simulink model "sfcndemo_port_triggered"  (Simulink 6.0)
settings: Solver=FixedStepDiscrete  SolverMode=SingleTasking  StartTime=0.0  StopTime=10.0  RelTol=1e-3
settings Model: Creator=The MathWorks Inc.  LastModifiedBy=batserve  ExtModeAutoUpdateStatusClock=off
settings OptimizationCC: BooleanDataType=off  InlineInvariantSignals=off
settings DebuggingCC: CheckExecutionContextPreStartOutputMsg=on  CheckExecutionContextRuntimeOutputMsg=on  SolverPrmCheckMsg=none
settings HardwareCC: TargetUnknown=on

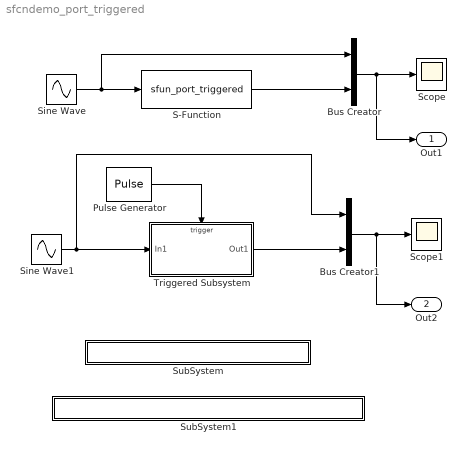
== system sfcndemo_port_triggered ==
  Bus Creator : BusCreator  DialogController=Simulink.DDGSource_Bus  Inputs=2
  Bus Creator1 : BusCreator  DialogController=Simulink.DDGSource_Bus  Inputs=2
  Pulse Generator : DiscretePulseGenerator  PulseType=Time based  PulseWidth=50
  S-Function : S-Function  FunctionName=sfun_port_triggered  Parameters=10
  Scope : Scope
  Scope1 : Scope
  Sine Wave : Sin  SampleTime=0.1
  Sine Wave1 : Sin  SampleTime=0
  SubSystem : Subsystem  PropExecContextAcrossSSBoundary=on
      settings: OpenFcn=edit(fullfile(matlabroot,'simulink','src','sfun_port_triggered.c'))
      mask Display: disp('matlabroot\simulink\src\sfun_port_triggered.c');
  SubSystem1 : Subsystem  PropExecContextAcrossSSBoundary=on
      settings: OpenFcn=edit(fullfile(matlabroot,'toolbox','simulink','blocks','tlc_c','sfun_port_triggered.tlc'))
      mask Display: disp('matlabroot\toolbox\simulink\blocks\tlc_c\sfun_port_triggered.tlc');
  Triggered Subsystem : Subsystem  TreatAsAtomicUnit=on  PropExecContextAcrossSSBoundary=on
  Out1 : Outport
  Out2 : Outport  Port=2
  wires:
  Pulse Generator/1 -> Triggered Subsystem/Trigger
  Sine Wave/1 -> S-Function/1, Bus Creator/1
  S-Function/1 -> Bus Creator/2
  Bus Creator/1 -> Scope/1, Out1/1
  Bus Creator1/1 -> Scope1/1, Out2/1
  Sine Wave1/1 -> Triggered Subsystem/1(In1), Bus Creator1/1
  Triggered Subsystem/1(Out1) -> Bus Creator1/2

== system sfcndemo_port_triggered/SubSystem ==

== system sfcndemo_port_triggered/SubSystem1 ==

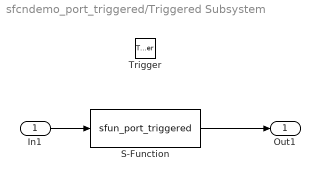
== system sfcndemo_port_triggered/Triggered Subsystem ==
  In1 : Inport  Port=1  LatchInput=off
  Trigger : TriggerPort
  S-Function : S-Function  FunctionName=sfun_port_triggered  Parameters=2
  Out1 : Outport
  wires:
  In1/1 -> S-Function/1
  S-Function/1 -> Out1/1
